simulink model "Tasks"  (R2024b)
settings: Solver=VariableStepAuto  StartTime=0.0  StopTime=3  RelTol=1e-3
model workspace (MATLAB code in the model file):
  | Ke = (2.53*10^(-3))*60/(2*pi); %V/(rad/s) Back EMF constant
  | Km = 24.2*10^(-3); %Nm/A    torque constant
  | L = 73*10^(-6); %H Terminal induction
  | R = 0.22; %ohm Terminal resictance
  | V = 24; %V Nominal supply voltage
  | J = 130*10^(-7);%kgm^2 %rotor inertia
  | frT = (7.72*10^(-7))*60/(2*pi); %Nm/(rad/s)  Friction torque dynamic
  | frTs=4.96e-3; %Nm Friction torque static
  | taum=4.9e-3; %Mechanical time constant
  | Mh=2635e-3; %Stall torqe Nm
  | I0=0.527; %no load current A
  | RADps_to_rpm=60/(2*pi);
  | RT=148e-3; %Rated torqe Nm
  | Rn=9650; %RPM rated speed
  | Rnnl=9700; %RPM rated speed no load
  | Mmaxout=55; %Max output torq
  | n=Mmaxout/Mh;
  | n1=n^0.5;
  | n2=n^0.5;
  | Jg1=6.5e-8;
  | Jg2=5.3e-8;
  | Jg=Jg1+(Jg2/(n1^2));
  | dj=1.5; %Nms/rad
  | 
  | dt=1.5; %Nms/rad
  | Kt=739; %Nm/rad
  | output_shaft_legth=(7.042+13.1+58)*(10^-3); %fyrkantstapp not included
  | avrage_diameter_output_shaft=(((24.5*10)+(19.6*11)+((58-19.6-24.5)*14)+(13.1*19.6)+(27.7*7.042))*(10^-6))/(output_shaft_legth); %fyrkantstapp not included.
  | input_shaft_solid_legth= (40.3-14)*10^-3;
  | avrage_diameter_input_solid_shaft= (((40.3-16.2)*5.9+(16.2-14)*11)*10^-6)/avrage_diameter_output_shaft;
  | input_shaft_hollow_legth=14e-3;
  | avrage_Odiameter_input_hollow_shaft=11e-3;
  | avrage_idiameter_input_hollow_shaft=8e-3;
  | Steel_density=7850; %kg/m^3
  | output_shaft_inertia=(Steel_density*output_shaft_legth*pi*((avrage_diameter_output_shaft/2)^4))/2;
  | input_shaft_solid_inertia=(Steel_density*input_shaft_solid_legth*pi*((avrage_diameter_input_solid_shaft/2)^4))/2;
  | input_shaft_hollow_inertia=(Steel_density*input_shaft_hollow_legth*pi*((avrage_Odiameter_input_hollow_shaft^2/4)-(avrage_idiameter_input_hollow_shaft^2/4)))*(((avrage_idiameter_input_hollow_shaft/2)^2)+((avrage_Odiameter_input_hollow_shaft/2)^2))/2;
  | input_shaft_inertia=input_shaft_hollow_inertia+input_shaft_solid_inertia;
  | Jin=input_shaft_inertia;
  | Jout=output_shaft_inertia;
  | J1=Jg+Jin+J;
  | J2=Jout;
  | A_Task6 =  [0, 0, 1, 0;
  |             0, 0, 0, 1;
  |             -Kt/(J1*n^2), Kt/(n*J1) , -(((dt/n^2)+(frT)+(Km*Ke/R))/J1),dt/(J1*n);
  |             Kt/(J2*n), -(Kt)/J2,dt/(n*J2), -(dj+dt)/J2];
  | B_Task6 = [0;
  |            0;
  |            Km/(R*J1);
  |            0];
  | C_Task6 = eye(4);
  | D_Task6 = [0;0;0;0];
  | 
  | 
  | 
  | Ks=4;%N/m
  | 
  | A_Task8 =  [0, 0, 1, 0;
  |             0, 0, 0, 1;
  |             -Kt/(J1*n^2), Kt/(n*J1) , -(((dt/n^2)+(frT)+(Km*Ke/R))/J1),dt/(J1*n);
  |             Kt/(J2*n), -(Kt+Ks)/J2,dt/(n*J2), -(dj+dt)/J2];
  | B_Task8 = [0;
  |            0;
  |            Km/(R*J1);
  |            0];
  | C_Task8 = eye(4);
  | D_Task8 = [0;0;0;0];
  | T=25;
  | Wtarget=3;
  | 
  | 
  | P=1.25e-3;%m
  | E=200e9; %Pa
  | Kj=Ks;
  | L0=100e-3; %m
  | sigmay=640e6; %Pa
  | %TargetT=(2*pi*L0*Kj*sigmay/(P*E));
  | r=4e-3; %m
  | Fy=pi*(r^2)*sigmay*10^6; %N
  | my=0.1;%-
  | Tmy=Fy*my*r; %Nm
  | thetay=(sigmay/((P/L0)*E))/(2*pi); %rad
  | Ftheta=(P/L0)*E*pi*(r^2)*2*pi*thetay*10^6; %F as a function of theta
  | Ty=Ks*thetay; %Nm
  | TargetT=Ty+Tmy; %Nm
  | 
  | 
  | Kpf=3/2.98;
undefined symbols (not defined in the file): sigbuilder_block
libraries: fl_lib x68, nesl_utility x18, slpidlib x5, sm_lib x4
(part 1 of 2)
settings Model: ParameterArgumentNames=A_Task6,A_Task8,B_Task6,B_Task8,C_Task6,C_Task8,D_Task6,D_Task8,I0,J,J1,J2,Jg,Jg1,Jg2,Jin,Jout,Ke,Km,Ks,Kt,L,Mh,Mmaxout,R,RADps_to_rpm,RT,Rn,Rnnl,Steel_density,T,V,Wtarget,avrage_Odiameter_input_hollow_shaft,avrage_diameter_input_solid_shaft,avrage_diameter_output_shaft,avrage_idiameter_input_hollow_shaft,dj,dt,frT,frTs,input_shaft_hollow_inertia,input_shaft_hollow_legth,input_shaft_inertia,input_shaft_solid_inertia,input_shaft_solid_legth,n,n1,n2,output_shaft_inertia,output_shaft_legth,taum  Creator=Johki  LastModifiedBy=chienh1

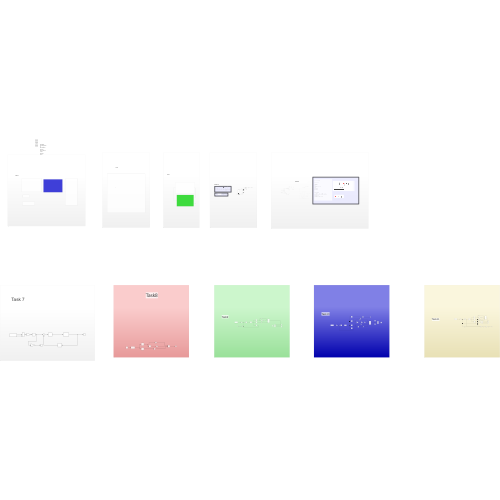
[thumbnail: Simulink's stored preview of the top-level diagram]
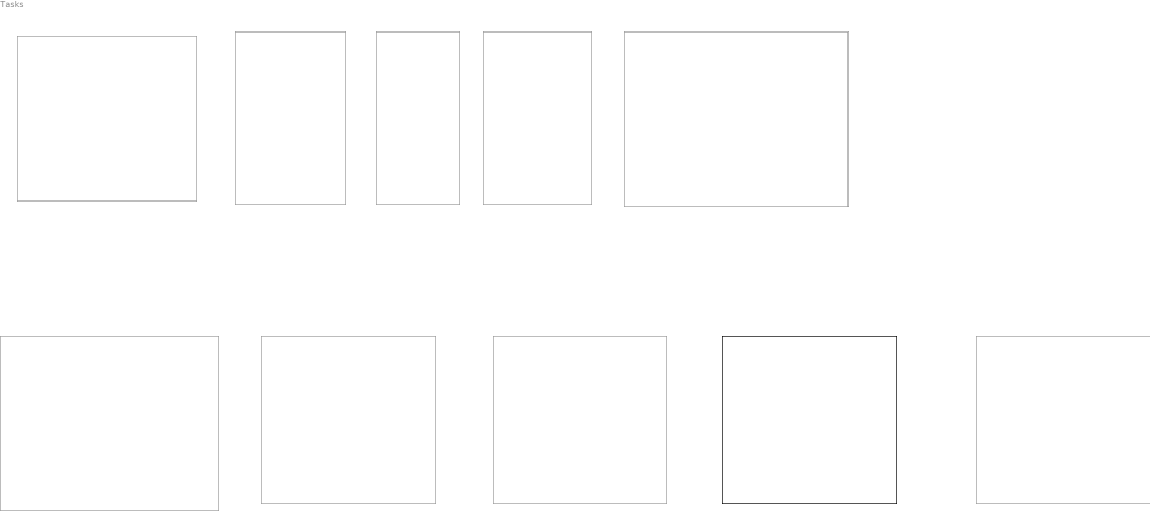
== system Tasks ==
  note: 2024-09-24:
      | Done: Repport so far
      | Start: Task9-11
      |
      | 2024-10-1
      | Done: Task9-11
      | Finnish
      |
      | 2024-10-7
      | "Done"
  note: 1: 8 points,
      | 2: 4 points,
      | 3: 4 points,
      | 4: 6 points,
      | 5: 2 points,
      | 6: 16 points,
      | 7: 6 points,
      | 8: 6 points,
      | 9: 8 points,
      | 10: 6 points,
      | 11: 4 points .
  Subsystem : Subsystem  Commented=on
  Subsystem1 : Subsystem  Commented=on
  Subsystem2 : Subsystem  Commented=on
  Subsystem3 : Subsystem  Commented=on
  Subsystem4 : Subsystem  Commented=on
  Subsystem5 : Subsystem  Commented=on
  Subsystem6 : Subsystem  Commented=on
  Subsystem7 : Subsystem
  Subsystem8 : Subsystem  Commented=on
  "Task6 " : Subsystem  Commented=on

== system Tasks/Subsystem ==
  note: Task 3
  Block diagram : Subsystem
  PI controller : Subsystem
  Terminator : Terminator
  wires:
  Block diagram/1(W) -> PI controller/1(ang velocity)
  PI controller/1(V) -> Block diagram/1(V)
  Block diagram/2(rpm) -> Terminator/1  "RPM_Block_dig"

== system Tasks/Subsystem1 ==
  note: Task 1
  Block diagram1 : Subsystem  Commented=on
  "SD " : Subsystem  Commented=on
  "Simscape " : Subsystem  Commented=on
  Simulink Model via State-Space Representation : Subsystem  Commented=on
  "Simulink Model via Transfer Function " : Subsystem  Commented=on

== system Tasks/Subsystem2 ==
  note: Task 2
  Subsystem5 : Subsystem
  Terminator3 : Terminator

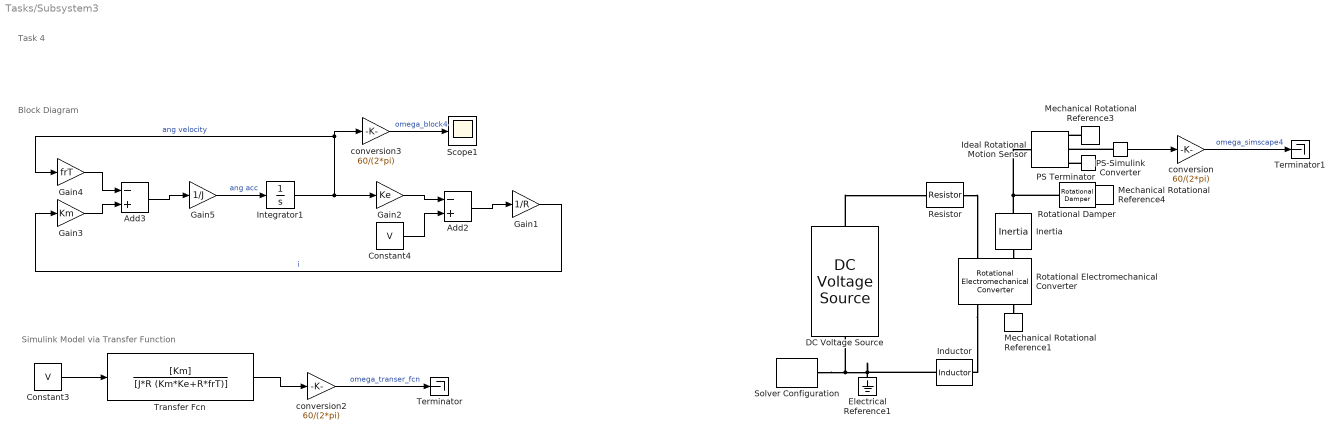
== system Tasks/Subsystem3 ==
  note: Block Diagram
  note: Simulink Model via Transfer Function
  note: Task 4
  Add2 : Sum  Inputs=-+
  Add3 : Sum  Inputs=-+
  Constant3 : Constant  Value=V
  Constant4 : Constant  Value=V
  DC Voltage Source : fl_lib/Electrical/Electrical Sources/DC Voltage Source  v0=V V
  Electrical Reference1 : fl_lib/Electrical/Electrical Elements/Electrical Reference
  Gain1 : Gain  Gain=1/R
  Gain2 : Gain  Gain=Ke
  Gain3 : Gain  Gain=Km
  Gain4 : Gain  Gain=frT
  Gain5 : Gain  Gain=1/J
  Ideal Rotational Motion Sensor : fl_lib/Mechanical/Mechanical Sensors/Ideal Rotational Motion Sensor  reference=foundation.enum.MeasurementReference.difference  acceleration_port=false  velocity_port=true  position_port=true  wrap_angle=simscape.enum.onoff.off  offset=0 rad
  Inductor : fl_lib/Electrical/Electrical Elements/Inductor  l=L H  r=0 Ohm  g=0 1/Ohm  i_specify=off  i_priority=None  i=0 A  i_nominal_specify=off  i_nominal_value=1  i_nominal_unit=A  v_specify=off  v_priority=None  v=0 V  v_nominal_specify=off  v_nominal_value=1  v_nominal_unit=V  i_L_specify=off  i_L_priority=High  i_L=0 A  i_L_nominal_specify=off  i_L_nominal_value=1  i_L_nominal_unit=A
  Inertia : fl_lib/Mechanical/Rotational Elements/Inertia  inertia=J kg*m^2  num_ports=foundation.enum.numPorts2.two  w_specify=off  w_priority=High  w=0 rad/s  w_nominal_specify=off  w_nominal_value=1  w_nominal_unit=rad/s  t_specify=off  t_priority=None  t=0 N*m  t_nominal_specify=off  t_nominal_value=1  t_nominal_unit=N*m
      settings: InternalSimscapePortConfiguration="{\"Bottom\":[],\"Left\":[{\"id\":\"I\",\"label\":\"\",\"type\":\"foundation.mechanical.rotational.rotational\"}],\"Right\":[{\"id\":\"J\",\"label\":\"\",\"type\":\"foundation.mechanical.rotational.rotational\"}],\"Top\":[]}"
  Integrator1 : Integrator
  Mechanical Rotational Reference1 : fl_lib/Mechanical/Rotational Elements/Mechanical Rotational Reference
  Mechanical Rotational Reference3 : fl_lib/Mechanical/Rotational Elements/Mechanical Rotational Reference
  Mechanical Rotational Reference4 : fl_lib/Mechanical/Rotational Elements/Mechanical Rotational Reference
  PS Terminator : fl_lib/Physical Signals/Sinks/PS Terminator
  PS-Simulink Converter : nesl_utility/PS-Simulink Converter  PhysicalDomain=network_engine_domain  SubClassName=ps_output  LeftPortType=input  RightPortType=output  PseudoPeriodic=off  Frequencies=[]  VectorFormat=inherit  Unit=inherit  AffineConversion=off
  Resistor : fl_lib/Electrical/Electrical Elements/Resistor  R=R Ohm  i_specify=off  i_priority=None  i=0 A  i_nominal_specify=off  i_nominal_value=1  i_nominal_unit=A  v_specify=off  v_priority=None  v=0 V  v_nominal_specify=off  v_nominal_value=1  v_nominal_unit=V
  Rotational Electromechanical Converter : fl_lib/Electrical/Electrical Elements/Rotational Electromechanical Converter  K=Ke V*s/rad  i_specify=off  i_priority=None  i=0 A  i_nominal_specify=off  i_nominal_value=1  i_nominal_unit=A  v_specify=off  v_priority=None  v=0 V  v_nominal_specify=off  v_nominal_value=1  v_nominal_unit=V  t_specify=off  t_priority=None  t=0 N*m  t_nominal_specify=off  t_nominal_value=1  t_nominal_unit=N*m  w_specify=on  w_priority=None  w=0 rad/s  w_nominal_specify=off  w_nominal_value=1  w_nominal_unit=rad/s
  Rotational Damper : fl_lib/Mechanical/Rotational Elements/Rotational Damper  D=frT N*m*s/rad  w_specify=off  w_priority=None  w=0 rad/s  w_nominal_specify=off  w_nominal_value=1  w_nominal_unit=rad/s  t_specify=off  t_priority=None  t=0 N*m  t_nominal_specify=off  t_nominal_value=1  t_nominal_unit=N*m
  Scope1 : Scope
  Solver Configuration : nesl_utility/Solver Configuration  PhysicalDomain=network_engine_domain  SubClassName=solver  LeftPortType=input  RightPortType=generic  Tones=[]  Harmonics=[]  SimulateNoise=off  Profile=off  UseLocalSampling=off  EnableSwitchedLinearOptims=on  FrequencyDomain=off  UseCCode=off  RelTol=0.001  AbsTol=0.001  MinStep=1e-09  ToWorkspace=off  RevertToSquareIcSolve=off  NumHomotopyIterations=100  PhasorMode=off  PhasorModeNumHarmonics=1  ConsistencySolver=NEWTON_FTOL  IndexReductionMethod=DerivativeReplacement  DoDC=off  ResidualTolerance=1e-09  ConsistencyTolSource=GLOBAL  ConsistencyAbsTol=0.001  ConsistencyRelTol=0.001  ConsistencyTolFactor=0.001  UseLocalSolver=off  LocalSolverChoice=NE_BACKWARD_EULER_ADVANCER  ResolveIndetEquations=on  FunctionEvalNumThread=1  LocalSolverSampleTime=0.001  DoFixedCost=off  MaxNonlinIter=3  MaxModeIter=2  ComputeImpulses=off  ImpulseIterations=2  LinearAlgebra=auto  LinearAlgebraNumThread=0  EquationFormulation=NE_TIME_EF  DelaysMemoryBudget=1024  AutomaticFiltering=on  FilteringTimeConstant=0.001  PartitionStorageMethod=AS_NEEDED  PartitionMemoryBudget=1024  PartitionMethod=ROBUST  MultibodyUseLocalSolver=off  MultibodyLocalSolverChoice=ODE1  MultibodyLocalSolverSampleTime=0.001
  Terminator : Terminator
  Terminator1 : Terminator
  Transfer Fcn : TransferFcn  Numerator=[Km]  Denominator=[J*R (Km*Ke+R*frT)]
  conversion : Gain  Gain=60/(2*pi)
  conversion2 : Gain  Gain=60/(2*pi)
  conversion3 : Gain  Gain=60/(2*pi)
  wires:
  Constant3/1 -> Transfer Fcn/1
  Transfer Fcn/1 -> conversion2/1
  conversion2/1 -> Terminator/1  "omega_transer_fcn"
  Gain2/1 -> Add2/1
  Add2/1 -> Gain1/1
  Gain1/1 -> Gain3/1  "i"
  Gain4/1 -> Add3/1
  Integrator1/1 -> conversion3/1, Gain4/1, Gain2/1  "ang velocity"
  Add3/1 -> Gain5/1
  Gain5/1 -> Integrator1/1  "ang acc"
  Constant4/1 -> Add2/2
  conversion3/1 -> Scope1/1  "omega_block4"
  Gain3/1 -> Add3/2
  conversion/1 -> Terminator1/1  "omega_simscape4"
  PS-Simulink Converter/1 -> conversion/1
  connections:
  DC Voltage Source/RConn1 -- Solver Configuration/RConn1 -- Inductor/RConn1 -- Electrical Reference1/LConn1
  Inertia/LConn1 -- Rotational Damper/LConn1 -- Ideal Rotational Motion Sensor/LConn1
  DC Voltage Source/LConn1 -- Resistor/LConn1
  PS-Simulink Converter/LConn1 -- Ideal Rotational Motion Sensor/RConn2
  Inertia/RConn1 -- Rotational Electromechanical Converter/LConn2
  Rotational Electromechanical Converter/RConn1 -- Inductor/LConn1
  Mechanical Rotational Reference4/LConn1 -- Rotational Damper/RConn1
  Rotational Electromechanical Converter/RConn2 -- Mechanical Rotational Reference1/LConn1
  Mechanical Rotational Reference3/LConn1 -- Ideal Rotational Motion Sensor/RConn1
  PS Terminator/LConn1 -- Ideal Rotational Motion Sensor/RConn3
  Resistor/RConn1 -- Rotational Electromechanical Converter/LConn1

== system Tasks/Subsystem4 ==
  note: Task 7
  Acceleration ref. : Subsystem  Tag=STV Subsys  LoadFcn=sigbuilder_block('load');  StartFcn=sigbuilder_block('start');  StopFcn=sigbuilder_block('stop');  ClipboardFcn=sigbuilder_block('clipboard');  mask(Sigbuilder block){tuvar=[0:10]}
      mask help: Sigbuilder GUI
      mask init:
      | if ~strcmp(get_param(bdroot(gcbh),'SimulationStatus'),'stopped') tuvar = sigbuilder_block('maskInit'); end
      settings: CopyFcn=sigbuilder_block('copy');  DeleteFcn=sigbuilder_block('delete');  ModelCloseFcn=sigbuilder_block('modelClose');  PreSaveFcn=sigbuilder_block('preSave');  PauseFcn=sigbuilder_block('pause')  ContinueFcn=sigbuilder_block('continue')  NameChangeFcn=sigbuilder_block('namechange');  OpenFcn=sigbuilder_block('open',[214.5 118 550.5 362 ]);  CloseFcn=sigbuilder_block('close');
      mask Display: plot(0, 0, 100, 100,[2, 2, 32, 32, 2], [68, 8, 8, 68, 68],[32, 2], [38, 38], [32, 19, 2],[53, 60, 44], [32, 17, 17, 2],[16, 16, 31, 31]);txt = getActiveGroup(gcbh);text(2, 100, txt,'verticalAlignment', 'top');
  PID Controller : slpidlib/PID Controller  Controller=PI  Form=Parallel  TimeDomain=Continuous-time  UseExternalTs=off  SampleTime=-1  IntegratorMethod=Forward Euler  FilterMethod=Forward Euler  ControllerParametersSource=internal  P=1.2  I=51  UseKiTs=off  D=0  UseExternalDerivativeSource=off  N=100  UseFilter=on  TunerSelectOption=Transfer Function Based (PID Tuner App)  InitialConditionSource=internal  InitialConditionForIntegrator=0  InitialConditionForFilter=0  DifferentiatorICPrevScaledInput=0  ExternalReset=none  TrackingMode=off  Kt=1  LimitOutput=off  SatLimitsSource=internal  UpperSaturationLimit=24  LowerSaturationLimit=0  LinearizeAsGain=on  AntiWindupMode=none  Kb=1  LimitIntegrator=off  UpperIntegratorSaturationLimit=inf  LowerIntegratorSaturationLimit=-inf  POutMin=[]  POutMax=[]  IOutMin=[]  IOutMax=[]  DOutMin=[]  DOutMax=[]  NOutMin=[]  NOutMax=[]  SumOutMin=[]  SumOutMax=[]  SaturationOutMin=[]  SaturationOutMax=[]  PParamMin=[]  PParamMax=[]  IParamMin=[]  IParamMax=[]  DParamMin=[]  DParamMax=[]  NParamMin=[]  NParamMax=[]  KbParamMin=[]  KbParamMax=[]  KtParamMin=[]  KtParamMax=[]  KbOutMin=[]  KbOutMax=[]  KtOutMin=[]  KtOutMax=[]  IntegratorOutMin=[]  IntegratorOutMax=[]  FilterOutMin=[]  FilterOutMax=[]  SumI1OutMin=[]  SumI1OutMax=[]  SumI2OutMin=[]  SumI2OutMax=[]  SumI3OutMin=[]  SumI3OutMax=[]  SumI4OutMin=[]  SumI4OutMax=[]  SumDOutMin=[]  SumDOutMax=[]  DifferentiatorOutMin=[]  DifferentiatorOutMax=[]  FilterDiffOutCoefMin=[]  FilterDiffOutCoefMax=[]  ReciprocalOutMin=[]  ReciprocalOutMax=[]  SumDenOutMin=[]  SumDenOutMax=[]  SumNumOutMin=[]  SumNumOutMax=[]  DivideOutMin=[]  DivideOutMax=[]  UdiffTsProdOutMin=[]  UdiffTsProdOutMax=[]  NTsProdOutMin=[]  NTsProdOutMax=[]  UintegralTsProdOutMin=[]  UintegralTsProdOutMax=[]  UngainTsProdOutMin=[]  UngainTsProdOutMax=[]  ClampingZeroOutDataTypeStr=Inherit: Inherit via back propagation  ClampingZeroOutMin=[]  ClampingZeroOutMax=[]  FilterDenConstantOutDataTypeStr=Inherit: Inherit via back propagation  FilterDenConstantOutMin=[]  FilterDenConstantOutMax=[]  PCopyOutDataTypeStr=Inherit: Inherit via back propagation  PCopyOutMin=[]  PCopyOutMax=[]  NCopyOutDataTypeStr=Inherit: Inherit via back propagation  NCopyOutMin=[]  NCopyOutMax=[]  IntegratorContinuousStateAttributes=''  IntegratorStateMustResolveToSignalObject=off  IntegratorRTWStateStorageClass=Auto  FilterContinuousStateAttributes=''  FilterStateMustResolveToSignalObject=off  FilterRTWStateStorageClass=Auto  ParallelPVariant=InternalParameters  IdealPVariant=Disabled  IVariant=InternalParameters  DVariant=Disabled  IntegratorVariant=Continuous  SatVariant=Disabled  AWVariant=Passthrough  PCopyVariant=Disabled  TRVariant=Disabled  FdbkBlocksVariant=Forward  IdealPFdbkVariant=Disabled  SatFdbkVariant=Disabled  DerivativeFilterVariant=Disabled  NVariant=Disabled  NCopyVariant=Disabled_SignalSpec  FilterICVariant=Disabled  IntegratorICVariant=InternalICs  ExternalResetVariant=Disabled  TRSumVariant=Passthrough  SumFdbkVariant=Disabled  SumVariant=Sum_PI  TsampFilterVariant=InternalTs  TsampNgainVariant=Passthrough  TsampIntegralVariant=Disabled_SignalSpec  ExternalSaturationOutDataTypeStr=Inherit: Same as second input  DerivativeSourceVariant=Disabled  PreIntVariant=InternalPreInt
  Scaling factor : Gain  Gain=15*n
  Scaling factor2 : Gain  Gain=1/n
  Selector : Selector  IndexMode=Zero-based  InputPortWidth=4  IndexOptions=Index vector (dialog)  Indices=2  OutputSizes=1
  State-Space : StateSpace  A=A_Task6  B=B_Task6  C=C_Task6  D=D_Task6  InitialCondition=0
  Sum : Sum  Inputs=|+-
  Sum2 : Sum  Inputs=|++
  Terminator : Terminator
  Vellocity ref : Integrator
  Y : Terminator
  wires:
  Sum2/1 -> Scaling factor/1
  Scaling factor/1 -> Vellocity ref/1
  Acceleration ref./1(Signal 1) -> Sum2/1
  Acceleration ref./2(Signal 2) -> Sum2/2
  State-Space/1 -> Y/1, Selector/1  "Y Task7"
  Sum/1 -> PID Controller/1
  Vellocity ref/1 -> Scaling factor2/1, Sum/1
  Selector/1 -> Sum/2  "phi1_dot_task7"
  PID Controller/1 -> State-Space/1  "V_Task7"
  Scaling factor2/1 -> Terminator/1  "Ref nut speed"

== system Tasks/Subsystem5 ==
  note: Task8
  24 V : Constant  Value=V
  Add : Sum  Inputs=+++
  Derivative : Derivative
  Gain : Gain  Gain=Ks
  Gain1 : Gain  Gain=dj
  Gain2 : Gain  Gain=J2
  Selector : Selector  InputPortWidth=4  IndexOptions=Index vector (dialog)  Indices=2  OutputSizes=1
  Selector1 : Selector  InputPortWidth=4  IndexOptions=Index vector (dialog)  Indices=4  OutputSizes=1
  State-Space : StateSpace  A=A_Task8  B=B_Task8  C=C_Task8  D=D_Task8  InitialCondition=0
  Terminator : Terminator
  wires:
  24 V/1 -> State-Space/1
  State-Space/1 -> Selector1/1, Selector/1  "States Task8"
  Selector/1 -> Gain/1  "phi 2"
  Selector1/1 -> Gain1/1, Derivative/1  "phi2 dot"
  Derivative/1 -> Gain2/1  "phi2 dotdot"
  Gain2/1 -> Add/2  "torsional inertia"
  Gain1/1 -> Add/1  "damping torque"
  Gain/1 -> Add/3  "torsional spring torque"
  Add/1 -> Terminator/1  "Total torque"

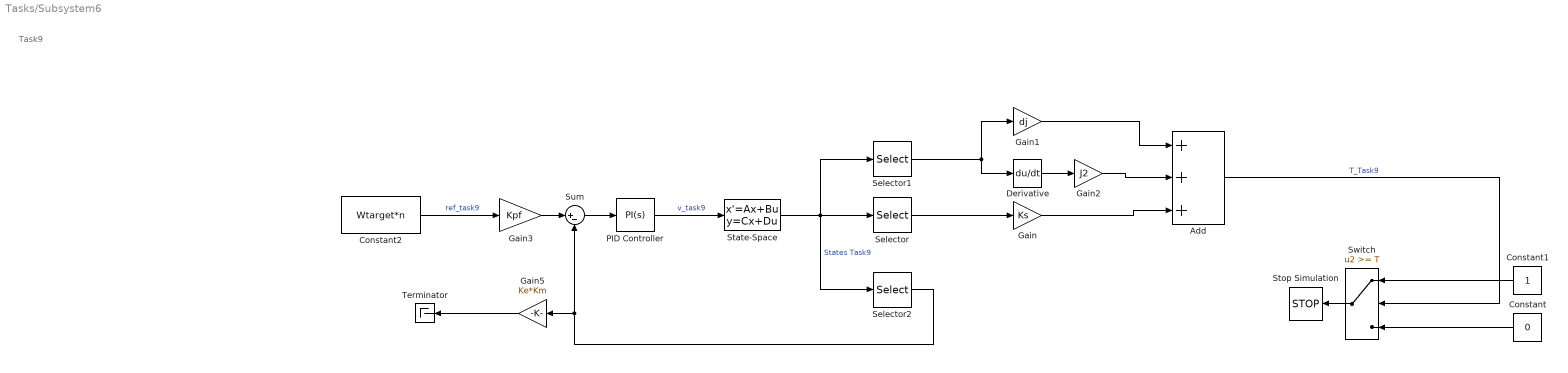
== system Tasks/Subsystem6 ==
  note: Task9
  Add : Sum  Inputs=+++
  Constant : Constant  Value=0
  Constant1 : Constant
  Constant2 : Constant  Value=Wtarget*n  VectorParams1D=off
  Derivative : Derivative
  Gain : Gain  Gain=Ks
  Gain1 : Gain  Gain=dj
  Gain2 : Gain  Gain=J2
  Gain3 : Gain  Gain=Kpf
  Gain5 : Gain  Gain=Ke*Km
  PID Controller : slpidlib/PID Controller  Controller=PI  Form=Parallel  TimeDomain=Continuous-time  UseExternalTs=off  SampleTime=-1  IntegratorMethod=Forward Euler  FilterMethod=Forward Euler  ControllerParametersSource=internal  P=24/(Wtarget*n*(Kpf))  I=1200  UseKiTs=off  D=0  UseExternalDerivativeSource=off  N=100  UseFilter=on  TunerSelectOption=Transfer Function Based (PID Tuner App)  InitialConditionSource=internal  InitialConditionForIntegrator=0  InitialConditionForFilter=0  DifferentiatorICPrevScaledInput=0  ExternalReset=none  TrackingMode=off  Kt=1  LimitOutput=off  SatLimitsSource=internal  UpperSaturationLimit=24  LowerSaturationLimit=0  LinearizeAsGain=on  AntiWindupMode=none  Kb=1  LimitIntegrator=off  UpperIntegratorSaturationLimit=inf  LowerIntegratorSaturationLimit=-inf  POutMin=[]  POutMax=[]  IOutMin=[]  IOutMax=[]  DOutMin=[]  DOutMax=[]  NOutMin=[]  NOutMax=[]  SumOutMin=[]  SumOutMax=[]  SaturationOutMin=[]  SaturationOutMax=[]  PParamMin=[]  PParamMax=[]  IParamMin=[]  IParamMax=[]  DParamMin=[]  DParamMax=[]  NParamMin=[]  NParamMax=[]  KbParamMin=[]  KbParamMax=[]  KtParamMin=[]  KtParamMax=[]  KbOutMin=[]  KbOutMax=[]  KtOutMin=[]  KtOutMax=[]  IntegratorOutMin=[]  IntegratorOutMax=[]  FilterOutMin=[]  FilterOutMax=[]  SumI1OutMin=[]  SumI1OutMax=[]  SumI2OutMin=[]  SumI2OutMax=[]  SumI3OutMin=[]  SumI3OutMax=[]  SumI4OutMin=[]  SumI4OutMax=[]  SumDOutMin=[]  SumDOutMax=[]  DifferentiatorOutMin=[]  DifferentiatorOutMax=[]  FilterDiffOutCoefMin=[]  FilterDiffOutCoefMax=[]  ReciprocalOutMin=[]  ReciprocalOutMax=[]  SumDenOutMin=[]  SumDenOutMax=[]  SumNumOutMin=[]  SumNumOutMax=[]  DivideOutMin=[]  DivideOutMax=[]  UdiffTsProdOutMin=[]  UdiffTsProdOutMax=[]  NTsProdOutMin=[]  NTsProdOutMax=[]  UintegralTsProdOutMin=[]  UintegralTsProdOutMax=[]  UngainTsProdOutMin=[]  UngainTsProdOutMax=[]  ClampingZeroOutDataTypeStr=Inherit: Inherit via back propagation  ClampingZeroOutMin=[]  ClampingZeroOutMax=[]  FilterDenConstantOutDataTypeStr=Inherit: Inherit via back propagation  FilterDenConstantOutMin=[]  FilterDenConstantOutMax=[]  PCopyOutDataTypeStr=Inherit: Inherit via back propagation  PCopyOutMin=[]  PCopyOutMax=[]  NCopyOutDataTypeStr=Inherit: Inherit via back propagation  NCopyOutMin=[]  NCopyOutMax=[]  IntegratorContinuousStateAttributes=''  IntegratorStateMustResolveToSignalObject=off  IntegratorRTWStateStorageClass=Auto  FilterContinuousStateAttributes=''  FilterStateMustResolveToSignalObject=off  FilterRTWStateStorageClass=Auto  ParallelPVariant=InternalParameters  IdealPVariant=Disabled  IVariant=InternalParameters  DVariant=Disabled  IntegratorVariant=Continuous  SatVariant=Disabled  AWVariant=Passthrough  PCopyVariant=Disabled  TRVariant=Disabled  FdbkBlocksVariant=Forward  IdealPFdbkVariant=Disabled  SatFdbkVariant=Disabled  DerivativeFilterVariant=Disabled  NVariant=Disabled  NCopyVariant=Disabled_SignalSpec  FilterICVariant=Disabled  IntegratorICVariant=InternalICs  ExternalResetVariant=Disabled  TRSumVariant=Passthrough  SumFdbkVariant=Disabled  SumVariant=Sum_PI  TsampFilterVariant=InternalTs  TsampNgainVariant=Passthrough  TsampIntegralVariant=Disabled_SignalSpec  ExternalSaturationOutDataTypeStr=Inherit: Same as second input  DerivativeSourceVariant=Disabled  PreIntVariant=InternalPreInt
  Selector : Selector  InputPortWidth=4  IndexOptions=Index vector (dialog)  Indices=2  OutputSizes=1
  Selector1 : Selector  InputPortWidth=4  IndexOptions=Index vector (dialog)  Indices=4  OutputSizes=1
  Selector2 : Selector  InputPortWidth=4  IndexOptions=Index vector (dialog)  Indices=3  OutputSizes=1
  State-Space : StateSpace  A=A_Task8  B=B_Task8  C=C_Task8  D=D_Task8  InitialCondition=0
  Stop Simulation : Stop
  Sum : Sum  Inputs=|+-
  Switch : Switch  Threshold=T  SaturateOnIntegerOverflow=off  InputSameDT=off
  Terminator : Terminator
  wires:
  Switch/1 -> Stop Simulation/1
  Constant/1 -> Switch/3
  Constant1/1 -> Switch/1
  Selector1/1 -> Derivative/1, Gain1/1
  Selector/1 -> Gain/1
  State-Space/1 -> Selector2/1, Selector/1, Selector1/1  "States Task9"
  Derivative/1 -> Gain2/1
  Add/1 -> Switch/2  "T_Task9"
  Gain/1 -> Add/3
  PID Controller/1 -> State-Space/1  "v_task9"
  Sum/1 -> PID Controller/1
  Selector2/1 -> Gain5/1, Sum/2
  Constant2/1 -> Gain3/1  "ref_task9"
  Gain3/1 -> Sum/1
  Gain2/1 -> Add/2
  Gain1/1 -> Add/1
  Gain5/1 -> Terminator/1

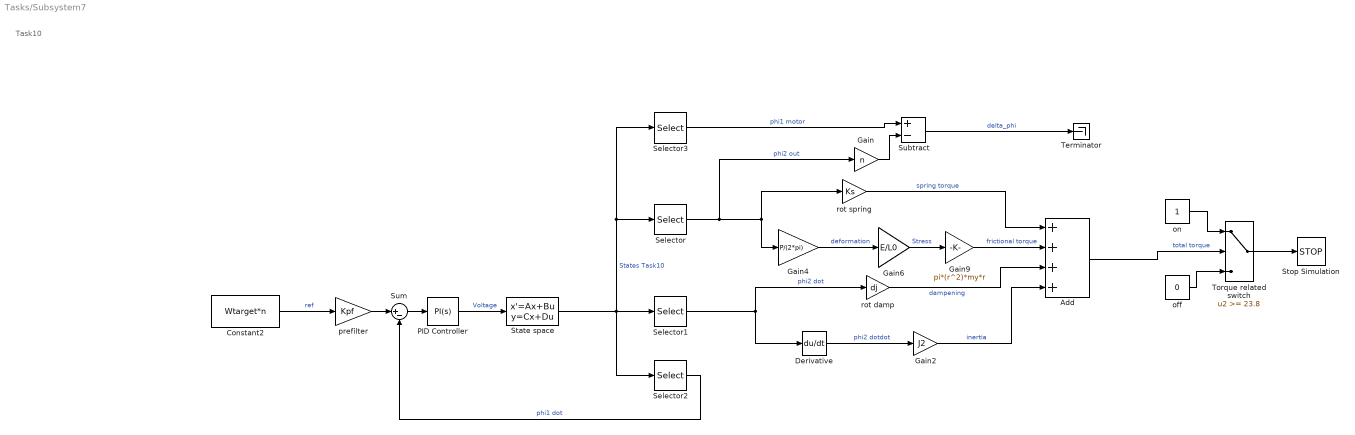
== system Tasks/Subsystem7 ==
  note: Task10
  Add : Sum  Inputs=++++
  Constant2 : Constant  Value=Wtarget*n  VectorParams1D=off
  Derivative : Derivative
  Gain : Gain  Gain=n
  Gain2 : Gain  Gain=J2
  Gain4 : Gain  Gain=P/(2*pi)
  Gain6 : Gain  Gain=E/L0
  Gain9 : Gain  Gain=pi*(r^2)*my*r
  PID Controller : slpidlib/PID Controller  Controller=PI  Form=Parallel  TimeDomain=Continuous-time  UseExternalTs=off  SampleTime=-1  IntegratorMethod=Forward Euler  FilterMethod=Forward Euler  ControllerParametersSource=internal  P=24/(Wtarget*n*Kpf)  I=1200  UseKiTs=off  D=0  UseExternalDerivativeSource=off  N=100  UseFilter=on  TunerSelectOption=Transfer Function Based (PID Tuner App)  InitialConditionSource=internal  InitialConditionForIntegrator=0  InitialConditionForFilter=0  DifferentiatorICPrevScaledInput=0  ExternalReset=none  TrackingMode=off  Kt=1  LimitOutput=off  SatLimitsSource=internal  UpperSaturationLimit=24  LowerSaturationLimit=0  LinearizeAsGain=on  AntiWindupMode=none  Kb=1  LimitIntegrator=off  UpperIntegratorSaturationLimit=inf  LowerIntegratorSaturationLimit=-inf  POutMin=[]  POutMax=[]  IOutMin=[]  IOutMax=[]  DOutMin=[]  DOutMax=[]  NOutMin=[]  NOutMax=[]  SumOutMin=[]  SumOutMax=[]  SaturationOutMin=[]  SaturationOutMax=[]  PParamMin=[]  PParamMax=[]  IParamMin=[]  IParamMax=[]  DParamMin=[]  DParamMax=[]  NParamMin=[]  NParamMax=[]  KbParamMin=[]  KbParamMax=[]  KtParamMin=[]  KtParamMax=[]  KbOutMin=[]  KbOutMax=[]  KtOutMin=[]  KtOutMax=[]  IntegratorOutMin=[]  IntegratorOutMax=[]  FilterOutMin=[]  FilterOutMax=[]  SumI1OutMin=[]  SumI1OutMax=[]  SumI2OutMin=[]  SumI2OutMax=[]  SumI3OutMin=[]  SumI3OutMax=[]  SumI4OutMin=[]  SumI4OutMax=[]  SumDOutMin=[]  SumDOutMax=[]  DifferentiatorOutMin=[]  DifferentiatorOutMax=[]  FilterDiffOutCoefMin=[]  FilterDiffOutCoefMax=[]  ReciprocalOutMin=[]  ReciprocalOutMax=[]  SumDenOutMin=[]  SumDenOutMax=[]  SumNumOutMin=[]  SumNumOutMax=[]  DivideOutMin=[]  DivideOutMax=[]  UdiffTsProdOutMin=[]  UdiffTsProdOutMax=[]  NTsProdOutMin=[]  NTsProdOutMax=[]  UintegralTsProdOutMin=[]  UintegralTsProdOutMax=[]  UngainTsProdOutMin=[]  UngainTsProdOutMax=[]  ClampingZeroOutDataTypeStr=Inherit: Inherit via back propagation  ClampingZeroOutMin=[]  ClampingZeroOutMax=[]  FilterDenConstantOutDataTypeStr=Inherit: Inherit via back propagation  FilterDenConstantOutMin=[]  FilterDenConstantOutMax=[]  PCopyOutDataTypeStr=Inherit: Inherit via back propagation  PCopyOutMin=[]  PCopyOutMax=[]  NCopyOutDataTypeStr=Inherit: Inherit via back propagation  NCopyOutMin=[]  NCopyOutMax=[]  IntegratorContinuousStateAttributes=''  IntegratorStateMustResolveToSignalObject=off  IntegratorRTWStateStorageClass=Auto  FilterContinuousStateAttributes=''  FilterStateMustResolveToSignalObject=off  FilterRTWStateStorageClass=Auto  ParallelPVariant=InternalParameters  IdealPVariant=Disabled  IVariant=InternalParameters  DVariant=Disabled  IntegratorVariant=Continuous  SatVariant=Disabled  AWVariant=Passthrough  PCopyVariant=Disabled  TRVariant=Disabled  FdbkBlocksVariant=Forward  IdealPFdbkVariant=Disabled  SatFdbkVariant=Disabled  DerivativeFilterVariant=Disabled  NVariant=Disabled  NCopyVariant=Disabled_SignalSpec  FilterICVariant=Disabled  IntegratorICVariant=InternalICs  ExternalResetVariant=Disabled  TRSumVariant=Passthrough  SumFdbkVariant=Disabled  SumVariant=Sum_PI  TsampFilterVariant=InternalTs  TsampNgainVariant=Passthrough  TsampIntegralVariant=Disabled_SignalSpec  ExternalSaturationOutDataTypeStr=Inherit: Same as second input  DerivativeSourceVariant=Disabled  PreIntVariant=InternalPreInt
  Selector : Selector  InputPortWidth=4  IndexOptions=Index vector (dialog)  Indices=2  OutputSizes=1
  Selector1 : Selector  InputPortWidth=4  IndexOptions=Index vector (dialog)  Indices=4  OutputSizes=1
  Selector2 : Selector  InputPortWidth=4  IndexOptions=Index vector (dialog)  Indices=3  OutputSizes=1
  Selector3 : Selector  InputPortWidth=4  IndexOptions=Index vector (dialog)  Indices=1  OutputSizes=1
  State space : StateSpace  A=A_Task8  B=B_Task8  C=C_Task8  D=D_Task8  InitialCondition=0
  Stop Simulation : Stop
  Subtract : Sum  Inputs=+-
  Sum : Sum  Inputs=|+-
  Terminator : Terminator
  Torque related switch : Switch  Threshold=23.8  SaturateOnIntegerOverflow=off  InputSameDT=off
  off : Constant  Value=0
  on : Constant
  prefilter : Gain  Gain=Kpf
  rot damp : Gain  Gain=dj
  rot spring : Gain  Gain=Ks
  wires:
  Selector2/1 -> Sum/2  "phi1 dot"
  prefilter/1 -> Sum/1
  Constant2/1 -> prefilter/1  "ref"
  Gain2/1 -> Add/4  "inertia"
  Torque related switch/1 -> Stop Simulation/1
  rot spring/1 -> Add/1  "spring torque"
  PID Controller/1 -> State space/1  "Voltage"
  Sum/1 -> PID Controller/1
  Add/1 -> Torque related switch/2  "total torque"
  State space/1 -> Selector3/1, Selector/1, Selector1/1, Selector2/1  "States Task10"
  Derivative/1 -> Gain2/1  "phi2 dotdot"
  off/1 -> Torque related switch/3
  on/1 -> Torque related switch/1
  rot damp/1 -> Add/3  "dampening"
  Selector1/1 -> rot damp/1, Derivative/1  "phi2 dot"
  Gain4/1 -> Gain6/1  "deformation"
  Gain6/1 -> Gain9/1  "Stress"
  Selector/1 -> Gain4/1, rot spring/1, Gain/1  "phi2 out"
  Gain9/1 -> Add/2  "frictional torque"
  Subtract/1 -> Terminator/1  "delta_phi"
  Selector3/1 -> Subtract/1  "phi1 motor"
  Gain/1 -> Subtract/2

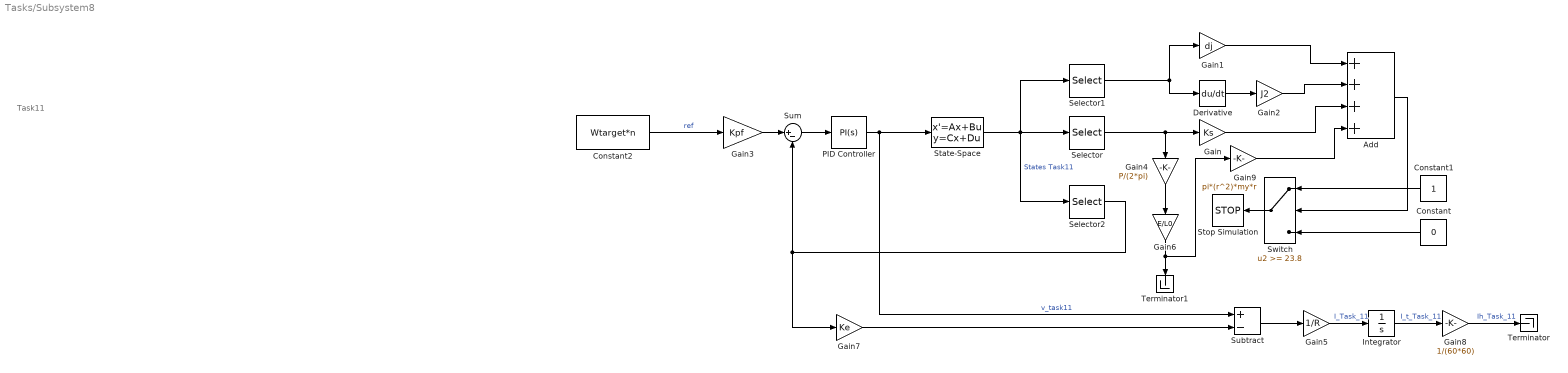
== system Tasks/Subsystem8 ==
  note: Task11
  Add : Sum  Inputs=++++
  Constant : Constant  Value=0
  Constant1 : Constant
  Constant2 : Constant  Value=Wtarget*n  VectorParams1D=off
  Derivative : Derivative
  Gain : Gain  Gain=Ks
  Gain1 : Gain  Gain=dj
  Gain2 : Gain  Gain=J2
  Gain3 : Gain  Gain=Kpf
  Gain4 : Gain  Gain=P/(2*pi)
  Gain5 : Gain  Gain=1/R
  Gain6 : Gain  Gain=E/L0
  Gain7 : Gain  Gain=Ke
  Gain8 : Gain  Gain=1/(60*60)
  Gain9 : Gain  Gain=pi*(r^2)*my*r
  Integrator : Integrator
  PID Controller : slpidlib/PID Controller  Controller=PI  Form=Parallel  TimeDomain=Continuous-time  UseExternalTs=off  SampleTime=-1  IntegratorMethod=Forward Euler  FilterMethod=Forward Euler  ControllerParametersSource=internal  P=24/(Wtarget*n*Kpf)  I=1200  UseKiTs=off  D=0  UseExternalDerivativeSource=off  N=100  UseFilter=on  TunerSelectOption=Transfer Function Based (PID Tuner App)  InitialConditionSource=internal  InitialConditionForIntegrator=0  InitialConditionForFilter=0  DifferentiatorICPrevScaledInput=0  ExternalReset=none  TrackingMode=off  Kt=1  LimitOutput=off  SatLimitsSource=internal  UpperSaturationLimit=24  LowerSaturationLimit=0  LinearizeAsGain=on  AntiWindupMode=none  Kb=1  LimitIntegrator=off  UpperIntegratorSaturationLimit=inf  LowerIntegratorSaturationLimit=-inf  POutMin=[]  POutMax=[]  IOutMin=[]  IOutMax=[]  DOutMin=[]  DOutMax=[]  NOutMin=[]  NOutMax=[]  SumOutMin=[]  SumOutMax=[]  SaturationOutMin=[]  SaturationOutMax=[]  PParamMin=[]  PParamMax=[]  IParamMin=[]  IParamMax=[]  DParamMin=[]  DParamMax=[]  NParamMin=[]  NParamMax=[]  KbParamMin=[]  KbParamMax=[]  KtParamMin=[]  KtParamMax=[]  KbOutMin=[]  KbOutMax=[]  KtOutMin=[]  KtOutMax=[]  IntegratorOutMin=[]  IntegratorOutMax=[]  FilterOutMin=[]  FilterOutMax=[]  SumI1OutMin=[]  SumI1OutMax=[]  SumI2OutMin=[]  SumI2OutMax=[]  SumI3OutMin=[]  SumI3OutMax=[]  SumI4OutMin=[]  SumI4OutMax=[]  SumDOutMin=[]  SumDOutMax=[]  DifferentiatorOutMin=[]  DifferentiatorOutMax=[]  FilterDiffOutCoefMin=[]  FilterDiffOutCoefMax=[]  ReciprocalOutMin=[]  ReciprocalOutMax=[]  SumDenOutMin=[]  SumDenOutMax=[]  SumNumOutMin=[]  SumNumOutMax=[]  DivideOutMin=[]  DivideOutMax=[]  UdiffTsProdOutMin=[]  UdiffTsProdOutMax=[]  NTsProdOutMin=[]  NTsProdOutMax=[]  UintegralTsProdOutMin=[]  UintegralTsProdOutMax=[]  UngainTsProdOutMin=[]  UngainTsProdOutMax=[]  ClampingZeroOutDataTypeStr=Inherit: Inherit via back propagation  ClampingZeroOutMin=[]  ClampingZeroOutMax=[]  FilterDenConstantOutDataTypeStr=Inherit: Inherit via back propagation  FilterDenConstantOutMin=[]  FilterDenConstantOutMax=[]  PCopyOutDataTypeStr=Inherit: Inherit via back propagation  PCopyOutMin=[]  PCopyOutMax=[]  NCopyOutDataTypeStr=Inherit: Inherit via back propagation  NCopyOutMin=[]  NCopyOutMax=[]  IntegratorContinuousStateAttributes=''  IntegratorStateMustResolveToSignalObject=off  IntegratorRTWStateStorageClass=Auto  FilterContinuousStateAttributes=''  FilterStateMustResolveToSignalObject=off  FilterRTWStateStorageClass=Auto  ParallelPVariant=InternalParameters  IdealPVariant=Disabled  IVariant=InternalParameters  DVariant=Disabled  IntegratorVariant=Continuous  SatVariant=Disabled  AWVariant=Passthrough  PCopyVariant=Disabled  TRVariant=Disabled  FdbkBlocksVariant=Forward  IdealPFdbkVariant=Disabled  SatFdbkVariant=Disabled  DerivativeFilterVariant=Disabled  NVariant=Disabled  NCopyVariant=Disabled_SignalSpec  FilterICVariant=Disabled  IntegratorICVariant=InternalICs  ExternalResetVariant=Disabled  TRSumVariant=Passthrough  SumFdbkVariant=Disabled  SumVariant=Sum_PI  TsampFilterVariant=InternalTs  TsampNgainVariant=Passthrough  TsampIntegralVariant=Disabled_SignalSpec  ExternalSaturationOutDataTypeStr=Inherit: Same as second input  DerivativeSourceVariant=Disabled  PreIntVariant=InternalPreInt
  Selector : Selector  InputPortWidth=4  IndexOptions=Index vector (dialog)  Indices=2  OutputSizes=1
  Selector1 : Selector  InputPortWidth=4  IndexOptions=Index vector (dialog)  Indices=4  OutputSizes=1
  Selector2 : Selector  InputPortWidth=4  IndexOptions=Index vector (dialog)  Indices=3  OutputSizes=1
  State-Space : StateSpace  A=A_Task8  B=B_Task8  C=C_Task8  D=D_Task8  InitialCondition=0
  Stop Simulation : Stop
  Subtract : Sum  Inputs=+-
  Sum : Sum  Inputs=|+-
  Switch : Switch  Threshold=23.8  SaturateOnIntegerOverflow=off  InputSameDT=off
  Terminator : Terminator
  Terminator1 : Terminator
  wires:
  Integrator/1 -> Gain8/1  "I_t_Task_11"
  Subtract/1 -> Gain5/1
  Gain8/1 -> Terminator/1  "Ih_Task_11"
  Gain9/1 -> Add/4
  Gain3/1 -> Sum/1
  Switch/1 -> Stop Simulation/1
  Selector2/1 -> Sum/2, Gain7/1
  Gain/1 -> Add/3
  Gain2/1 -> Add/2
  Gain4/1 -> Gain6/1
  Gain5/1 -> Integrator/1  "I_Task_11"
  Selector/1 -> Gain/1, Gain4/1
  Gain7/1 -> Subtract/2
  Constant1/1 -> Switch/1
  PID Controller/1 -> State-Space/1, Subtract/1  "v_task11"
  Gain1/1 -> Add/1
  Add/1 -> Switch/2
  State-Space/1 -> Selector2/1, Selector/1, Selector1/1  "States Task11"
  Derivative/1 -> Gain2/1
  Gain6/1 -> Gain9/1, Terminator1/1
  Constant/1 -> Switch/3
  Sum/1 -> PID Controller/1
  Selector1/1 -> Derivative/1, Gain1/1
  Constant2/1 -> Gain3/1  "ref"

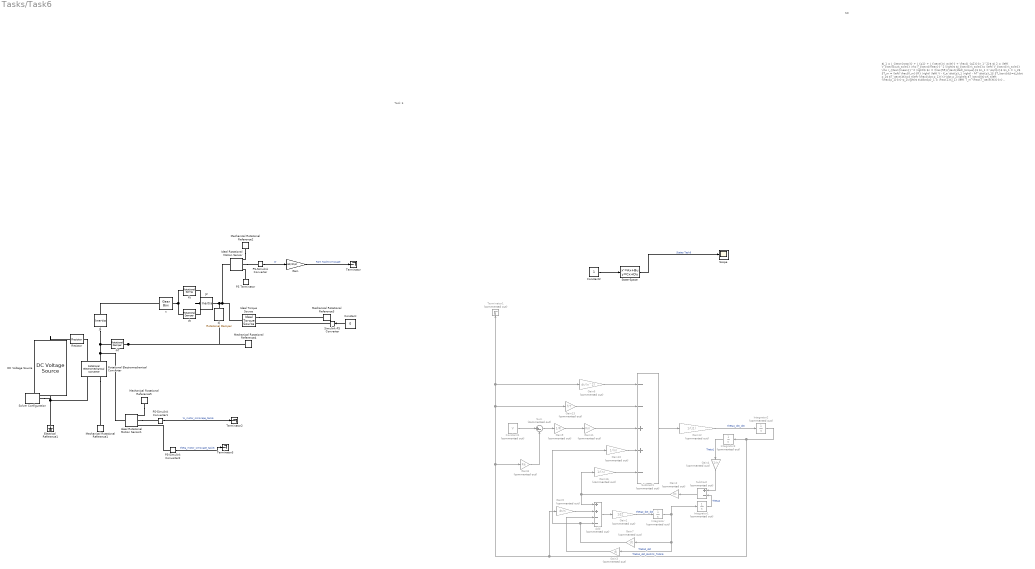
== system Tasks/Task6  ==
  note: $J_1 = J_{\text{rotor}} + J_{g1} + J_{\text{in\_axle}} + \frac{J_{g2}}{n_1^2}$
      | $J_2 = \left( V_{\text{out\_axle}} \rho r_{\text{mean}}^2 \right)$
      |
      | $J_{\text{in\_axle}}= \left( V_{\text{in\_axle}} \rho r_{\text{mean}}^2 \right)$
      |
      | $n = \frac{55}{\text{stall\_torque}}$
      | $n_1 = \sqrt{n}$
      | $n_1 = n_2$
      |
      | $T_m = \left( \frac{K_m}{R} \right) \left( V - K_e \dot{p}_1 \right) - frT \dot{p}_1$
      | $T_\text{dj}=d_j\dot p_2$
      | $T_\text{dt}=d_t\left (\frac{\dot p_1}{n}-\dot p_2\right)$
      | $T_\text{Kt}=K_t\left (\frac{p_1}{n}-p_2\right)$
      |
      | $\ddot{p}_1 = \frac{1}{J_1} \left( T_m -\frac{T_\text{Kt}}{n} -\frac{T_\text{dt}}{n}\right)$
      |
      | $\ddot{p}_1 = \frac{1}{J_1} \left( \frac{K_mV}{R} - \frac{K_t}{n^2}p_1 -\frac{K_t}{n} p_2 - \left(\frac{d_t}{n^2} -\frac{K_mK_e}{R}- frT\right)\dot{p}_1 +\frac{dt}{n}\dot{p}_2\right)$
      | $\ddot{p}_2 = \frac{1}{J_2} \left(T_\text{Kt} +T_\text{dt}-T_\text{dj}\right)$
      | $\ddot{p}_2 = \frac{1}{J_2} \left( K_t\frac{p_1}{n} - K_t p_2 +\frac{dt}{n}\dot{p}_1 - (d_j+d_t)\dot{p}_2\right)$
  note: Task 6
  note: SD
  Add : Sum  Commented=on  Inputs=++--
  Constant : Constant  Value=0
  Constant1 : Constant  Commented=on  Value=V
  Constant2 : Constant
  DC Voltage Source : fl_lib/Electrical/Electrical Sources/DC Voltage Source  v0=V V
  Electrical Reference1 : fl_lib/Electrical/Electrical Elements/Electrical Reference
  Gain : Gain  Gain=60/(2*pi)
  Gain1 : Gain  Commented=on  Gain=1/J2
  Gain10 : Gain  Commented=on  Gain=1/(n)
  Gain11 : Gain  Commented=on  Gain=Km
  Gain12 : Gain  Commented=on  Gain=1/(J1)
  Gain13 : Gain  Commented=on  Gain=frT
  Gain16 : Gain  Commented=on  Gain=1/(n)
  Gain2 : Gain  Commented=on  Gain=Kt
  Gain3 : Gain  Commented=on  Gain=dj
  Gain4 : Gain  Commented=on  Gain=1/n
  Gain5 : Gain  Commented=on  Gain=dt/n
  Gain6 : Gain  Commented=on  Gain=dt/(n^2)
  Gain7 : Gain  Commented=on  Gain=dt
  Gain8 : Gain  Commented=on  Gain=Ke
  Gain9 : Gain  Commented=on  Gain=1/R
  Ideal Rotational Motion Sensor : fl_lib/Mechanical/Mechanical Sensors/Ideal Rotational Motion Sensor  reference=foundation.enum.MeasurementReference.difference  acceleration_port=false  velocity_port=true  position_port=true  wrap_angle=simscape.enum.onoff.off  offset=0 rad
  Ideal Rotational Motion Sensor1 : fl_lib/Mechanical/Mechanical Sensors/Ideal Rotational Motion Sensor  reference=foundation.enum.MeasurementReference.difference  acceleration_port=false  velocity_port=true  position_port=true  wrap_angle=simscape.enum.onoff.off  offset=0 rad
  Ideal Torque Source : fl_lib/Mechanical/Mechanical Sources/Ideal Torque Source
  Integrator{,1..3} (4 alike) : Integrator  Commented=on
  J1 : fl_lib/Mechanical/Rotational Elements/Inertia  inertia=J1 kg*m^2  num_ports=foundation.enum.numPorts2.two  w_specify=off  w_priority=High  w=0 rad/s  w_nominal_specify=off  w_nominal_value=1  w_nominal_unit=rad/s  t_specify=off  t_priority=None  t=0 N*m  t_nominal_specify=off  t_nominal_value=1  t_nominal_unit=N*m
      settings: InternalSimscapePortConfiguration="{\"Bottom\":[],\"Left\":[{\"id\":\"I\",\"label\":\"\",\"type\":\"foundation.mechanical.rotational.rotational\"}],\"Right\":[{\"id\":\"J\",\"label\":\"\",\"type\":\"foundation.mechanical.rotational.rotational\"}],\"Top\":[]}"
  J2 : fl_lib/Mechanical/Rotational Elements/Inertia  inertia=J2 kg*m^2  num_ports=foundation.enum.numPorts2.two  w_specify=off  w_priority=High  w=0 rad/s  w_nominal_specify=off  w_nominal_value=1  w_nominal_unit=rad/s  t_specify=off  t_priority=None  t=0 N*m  t_nominal_specify=off  t_nominal_value=1  t_nominal_unit=N*m
      settings: InternalSimscapePortConfiguration="{\"Bottom\":[],\"Left\":[{\"id\":\"I\",\"label\":\"\",\"type\":\"foundation.mechanical.rotational.rotational\"}],\"Right\":[{\"id\":\"J\",\"label\":\"\",\"type\":\"foundation.mechanical.rotational.rotational\"}],\"Top\":[]}"
  Kt : fl_lib/Mechanical/Rotational Elements/Rotational Spring  spr_rate=Kt N*m/rad  w_specify=off  w_priority=None  w=0 rad/s  w_nominal_specify=off  w_nominal_value=1  w_nominal_unit=rad/s  t_specify=off  t_priority=None  t=0 N*m  t_nominal_specify=off  t_nominal_value=1  t_nominal_unit=N*m  phi_specify=off  phi_priority=High  phi=0 rad  phi_nominal_specify=off  phi_nominal_value=1  phi_nominal_unit=rad
  Mechanical Rotational Reference{1..5} (5 alike) : fl_lib/Mechanical/Rotational Elements/Mechanical Rotational Reference
  PS Terminator : fl_lib/Physical Signals/Sinks/PS Terminator
  PS-Simulink Converter : nesl_utility/PS-Simulink Converter  PhysicalDomain=network_engine_domain  SubClassName=ps_output  LeftPortType=input  RightPortType=output  PseudoPeriodic=off  Frequencies=[]  VectorFormat=inherit  Unit=inherit  AffineConversion=off
  PS-Simulink Converter1 : nesl_utility/PS-Simulink Converter  PhysicalDomain=network_engine_domain  SubClassName=ps_output  LeftPortType=input  RightPortType=output  PseudoPeriodic=off  Frequencies=[]  VectorFormat=inherit  Unit=inherit  AffineConversion=off
  PS-Simulink Converter2 : nesl_utility/PS-Simulink Converter  PhysicalDomain=network_engine_domain  SubClassName=ps_output  LeftPortType=input  RightPortType=output  PseudoPeriodic=off  Frequencies=[]  VectorFormat=inherit  Unit=inherit  AffineConversion=off
  Resistor : fl_lib/Electrical/Electrical Elements/Resistor  R=R Ohm  i_specify=off  i_priority=None  i=0 A  i_nominal_specify=off  i_nominal_value=1  i_nominal_unit=A  v_specify=off  v_priority=None  v=0 V  v_nominal_specify=off  v_nominal_value=1  v_nominal_unit=V
  Rotational Electromechanical Converter : fl_lib/Electrical/Electrical Elements/Rotational Electromechanical Converter  K=Ke V*s/rad  i_specify=off  i_priority=None  i=0 A  i_nominal_specify=off  i_nominal_value=1  i_nominal_unit=A  v_specify=off  v_priority=None  v=0 V  v_nominal_specify=off  v_nominal_value=1  v_nominal_unit=V  t_specify=off  t_priority=None  t=0 N*m  t_nominal_specify=off  t_nominal_value=1  t_nominal_unit=N*m  w_specify=on  w_priority=None  w=0 rad/s  w_nominal_specify=off  w_nominal_value=1  w_nominal_unit=rad/s
  Scope : Scope
  Simulink-PS Converter : nesl_utility/Simulink-PS Converter  PhysicalDomain=network_engine_domain  SubClassName=ps_input  LeftPortType=input  RightPortType=output  PseudoPeriodic=off  Frequencies=[]  NoiseDistribution=none  NoiseParameters=[]  Unit=1  AffineConversion=off  FilteringAndDerivatives=provide  SimscapeFilterOrder=1  InputFilterTimeConstant=0.001  UdotUserProvided=0
  Solver Configuration : nesl_utility/Solver Configuration  PhysicalDomain=network_engine_domain  SubClassName=solver  LeftPortType=input  RightPortType=generic  Tones=[]  Harmonics=[]  SimulateNoise=off  Profile=off  UseLocalSampling=off  EnableSwitchedLinearOptims=on  FrequencyDomain=off  UseCCode=off  RelTol=0.001  AbsTol=0.001  MinStep=1e-09  ToWorkspace=off  RevertToSquareIcSolve=off  NumHomotopyIterations=100  PhasorMode=off  PhasorModeNumHarmonics=1  ConsistencySolver=NEWTON_FTOL  IndexReductionMethod=DerivativeReplacement  DoDC=off  ResidualTolerance=1e-09  ConsistencyTolSource=GLOBAL  ConsistencyAbsTol=0.001  ConsistencyRelTol=0.001  ConsistencyTolFactor=0.001  UseLocalSolver=off  LocalSolverChoice=NE_BACKWARD_EULER_ADVANCER  ResolveIndetEquations=on  FunctionEvalNumThread=1  LocalSolverSampleTime=0.001  DoFixedCost=off  MaxNonlinIter=3  MaxModeIter=2  ComputeImpulses=off  ImpulseIterations=2  LinearAlgebra=auto  LinearAlgebraNumThread=0  EquationFormulation=NE_TIME_EF  DelaysMemoryBudget=1024  AutomaticFiltering=on  FilteringTimeConstant=0.001  PartitionStorageMethod=AS_NEEDED  PartitionMemoryBudget=1024  PartitionMethod=ROBUST  MultibodyUseLocalSolver=off  MultibodyLocalSolverChoice=ODE1  MultibodyLocalSolverSampleTime=0.001
  State-Space : StateSpace  A=A_Task6  B=B_Task6  C=C_Task6  D=D_Task6  InitialCondition=0
  Subtract : Sum  Commented=on  Inputs=+-
  Subtract1 : Sum  Commented=on  Inputs=--++-
  Sum : Sum  Commented=on  Inputs=|+-
  Terminator : Terminator
  Terminator1 : Terminator  Commented=on
  Terminator2 : Terminator
  Terminator3 : Terminator
  dj : fl_lib/Mechanical/Rotational Elements/Rotational Damper  D=dj N*m*s/rad  w_specify=off  w_priority=None  w=0 rad/s  w_nominal_specify=off  w_nominal_value=1  w_nominal_unit=rad/s  t_specify=off  t_priority=None  t=0 N*m  t_nominal_specify=off  t_nominal_value=1  t_nominal_unit=N*m
  dt : fl_lib/Mechanical/Rotational Elements/Rotational Damper  D=dt N*m*s/rad  w_specify=off  w_priority=None  w=0 rad/s  w_nominal_specify=off  w_nominal_value=1  w_nominal_unit=rad/s  t_specify=off  t_priority=None  t=0 N*m  t_nominal_specify=off  t_nominal_value=1  t_nominal_unit=N*m
  frT : fl_lib/Mechanical/Rotational Elements/Rotational Damper  D=frT N*m*s/rad  w_specify=off  w_priority=None  w=0 rad/s  w_nominal_specify=off  w_nominal_value=1  w_nominal_unit=rad/s  t_specify=off  t_priority=None  t=0 N*m  t_nominal_specify=off  t_nominal_value=1  t_nominal_unit=N*m
  n : fl_lib/Mechanical/Mechanisms/Gear Box  ratio=n  t_in_specify=off  t_in_priority=None  t_in=0 N*m  t_in_nominal_specify=off  t_in_nominal_value=1  t_in_nominal_unit=N*m  t_out_specify=off  t_out_priority=None  t_out=0 N*m  t_out_nominal_specify=off  t_out_nominal_value=1  t_out_nominal_unit=N*m
  wires:
  PS-Simulink Converter/1 -> Gain/1  "W"
  Gain/1 -> Terminator/1  "Rpm Task5 simscape"
  Constant/1 -> Simulink-PS Converter/1
  Gain4/1 -> Subtract/1
  Subtract/1 -> Gain2/1
  Gain16/1 -> Subtract1/5
  Gain12/1 -> Integrator2/1  "theta1_dot_dot"
  Add/1 -> Gain1/1
  Sum/1 -> Gain9/1
  Gain9/1 -> Gain11/1
  Integrator2/1 -> Gain5/1, Terminator1/1, Gain6/1, Gain13/1, Gain8/1, Integrator3/1  "Theta1_dot_BLOCK_TASK6"
  Integrator3/1 -> Gain4/1  "Theta1"
  Gain13/1 -> Subtract1/2
  Integrator1/1 -> Subtract/2  "Theta2"
  Subtract1/1 -> Gain12/1
  Integrator/1 -> Integrator1/1, Gain7/1, Gain3/1  "Theta2_dot"
  Gain11/1 -> Subtract1/3
  Constant1/1 -> Sum/1
  Gain3/1 -> Add/3
  Gain1/1 -> Integrator/1  "theta2_dot_dot"
  Gain8/1 -> Sum/2
  PS-Simulink Converter1/1 -> Terminator2/1  "W_motor_simscape_task6"
  Gain6/1 -> Subtract1/1
  Constant2/1 -> State-Space/1
  State-Space/1 -> Scope/1  "States Task6"
  PS-Simulink Converter2/1 -> Terminator3/1  "theta_motor_simscape_task6"
  Gain5/1 -> Add/2
  Gain7/1 -> Add/4, Gain10/1
  Gain2/1 -> Gain16/1, Add/1
  Gain10/1 -> Subtract1/4
  connections:
  Ideal Rotational Motion Sensor/RConn2 -- PS-Simulink Converter/LConn1
  Resistor/RConn1 -- Rotational Electromechanical Converter/LConn1
  Rotational Electromechanical Converter/RConn2 -- Mechanical Rotational Reference1/LConn1
  Ideal Torque Source/RConn2 -- Mechanical Rotational Reference3/LConn1
  frT/RConn1 -- Mechanical Rotational Reference4/LConn1 -- dj/RConn1
  PS Terminator/LConn1 -- Ideal Rotational Motion Sensor/RConn3
  DC Voltage Source/LConn1 -- Resistor/LConn1
  n/RConn1 -- dt/LConn1 -- Kt/LConn1
  J2/RConn1 -- dj/LConn1 -- Ideal Rotational Motion Sensor/LConn1 -- Ideal Torque Source/LConn1
  Simulink-PS Converter/RConn1 -- Ideal Torque Source/RConn1
  PS-Simulink Converter2/LConn1 -- Ideal Rotational Motion Sensor1/RConn3
  Ideal Rotational Motion Sensor1/RConn2 -- PS-Simulink Converter1/LConn1
  J2/LConn1 -- dt/RConn1 -- Kt/RConn1
  J1/LConn1 -- n/LConn1
  Rotational Electromechanical Converter/LConn2 -- Ideal Rotational Motion Sensor1/LConn1 -- frT/LConn1 -- J1/RConn1
  Electrical Reference1/LConn1 -- Rotational Electromechanical Converter/RConn1 -- Solver Configuration/RConn1 -- DC Voltage Source/RConn1
  Mechanical Rotational Reference2/LConn1 -- Ideal Rotational Motion Sensor/RConn1
  Mechanical Rotational Reference5/LConn1 -- Ideal Rotational Motion Sensor1/RConn1

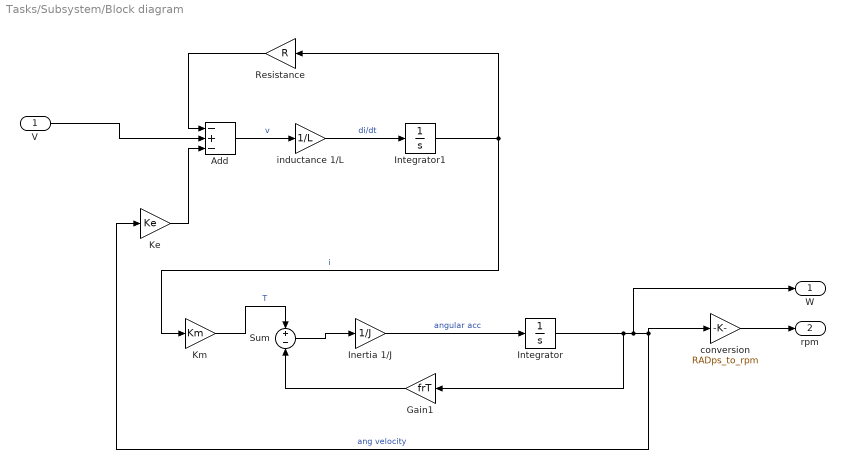
== system Tasks/Subsystem/Block diagram ==
  V : Inport
  Add : Sum  Inputs=-+-
  Gain1 : Gain  Gain=frT
  Inertia 1/J : Gain  Gain=1/J
  Integrator : Integrator
  Integrator1 : Integrator
  Ke : Gain  Gain=Ke
  Km : Gain  Gain=Km
  Resistance : Gain  Gain=R
  Sum : Sum  Inputs=+-
  conversion : Gain  Gain=RADps_to_rpm
  inductance 1/L : Gain  Gain=1/L
  W : Outport
  rpm : Outport  Port=2
  wires:
  Ke/1 -> Add/3
  Sum/1 -> Inertia 1/J/1
  inductance 1/L/1 -> Integrator1/1  "di/dt"
  Km/1 -> Sum/1  "T"
  Inertia 1/J/1 -> Integrator/1  "angular acc"
  Gain1/1 -> Sum/2
  Add/1 -> inductance 1/L/1  "v"
  Integrator1/1 -> Km/1, Resistance/1  "i"
  Integrator/1 -> conversion/1, Ke/1, W/1, Gain1/1  "ang velocity"
  Resistance/1 -> Add/1
  V/1 -> Add/2
  conversion/1 -> rpm/1

== system Tasks/Subsystem/PI controller ==
  note: Develop in Simulink an angular velocity PI controller for the DC-motor using the block-diagram model of the motor and show the resulting block diagram model. Assume that you can sense angular velocity and acceleration directly. Tune the controller to make a quick response without overshooting to an input reference step of 12 rad/s and make sure and demonstrate not to violate any voltage or current limitations of the motor. However, the starting current is allowed to be 500% of the rated current. Demonstrate the controller’s performance by time domain plots and state your controller settings
  ang velocity : Inport
  Step : Step  Time=0  After=12  SampleTime=0
  Sum1 : Sum  Inputs=+-
  Varying PID Controller : slpidlib/PID Controller  Controller=PI  Form=Parallel  TimeDomain=Continuous-time  UseExternalTs=off  SampleTime=-1  IntegratorMethod=Forward Euler  FilterMethod=Forward Euler  ControllerParametersSource=internal  P=0.218326262588512  I=6.46147954848858  UseKiTs=off  D=0  UseExternalDerivativeSource=off  N=100  UseFilter=on  TunerSelectOption=Transfer Function Based (PID Tuner App)  InitialConditionSource=internal  InitialConditionForIntegrator=0  InitialConditionForFilter=0  DifferentiatorICPrevScaledInput=0  ExternalReset=none  TrackingMode=off  Kt=1  LimitOutput=on  SatLimitsSource=internal  UpperSaturationLimit=V*1.2  LowerSaturationLimit=0  LinearizeAsGain=off  AntiWindupMode=none  Kb=1  LimitIntegrator=off  UpperIntegratorSaturationLimit=inf  LowerIntegratorSaturationLimit=-inf  POutMin=[]  POutMax=[]  IOutMin=[]  IOutMax=[]  DOutMin=[]  DOutMax=[]  NOutMin=[]  NOutMax=[]  SumOutMin=[]  SumOutMax=[]  SaturationOutMin=[]  SaturationOutMax=[]  PParamMin=[]  PParamMax=[]  IParamMin=[]  IParamMax=[]  DParamMin=[]  DParamMax=[]  NParamMin=[]  NParamMax=[]  KbParamMin=[]  KbParamMax=[]  KtParamMin=[]  KtParamMax=[]  KbOutMin=[]  KbOutMax=[]  KtOutMin=[]  KtOutMax=[]  IntegratorOutMin=[]  IntegratorOutMax=[]  FilterOutMin=[]  FilterOutMax=[]  SumI1OutMin=[]  SumI1OutMax=[]  SumI2OutMin=[]  SumI2OutMax=[]  SumI3OutMin=[]  SumI3OutMax=[]  SumI4OutMin=[]  SumI4OutMax=[]  SumDOutMin=[]  SumDOutMax=[]  DifferentiatorOutMin=[]  DifferentiatorOutMax=[]  FilterDiffOutCoefMin=[]  FilterDiffOutCoefMax=[]  ReciprocalOutMin=[]  ReciprocalOutMax=[]  SumDenOutMin=[]  SumDenOutMax=[]  SumNumOutMin=[]  SumNumOutMax=[]  DivideOutMin=[]  DivideOutMax=[]  UdiffTsProdOutMin=[]  UdiffTsProdOutMax=[]  NTsProdOutMin=[]  NTsProdOutMax=[]  UintegralTsProdOutMin=[]  UintegralTsProdOutMax=[]  UngainTsProdOutMin=[]  UngainTsProdOutMax=[]  ClampingZeroOutDataTypeStr=Inherit: Inherit via back propagation  ClampingZeroOutMin=[]  ClampingZeroOutMax=[]  FilterDenConstantOutDataTypeStr=Inherit: Inherit via back propagation  FilterDenConstantOutMin=[]  FilterDenConstantOutMax=[]  PCopyOutDataTypeStr=Inherit: Inherit via back propagation  PCopyOutMin=[]  PCopyOutMax=[]  NCopyOutDataTypeStr=Inherit: Inherit via back propagation  NCopyOutMin=[]  NCopyOutMax=[]  IntegratorContinuousStateAttributes=''  IntegratorStateMustResolveToSignalObject=off  IntegratorRTWStateStorageClass=Auto  FilterContinuousStateAttributes=''  FilterStateMustResolveToSignalObject=off  FilterRTWStateStorageClass=Auto  ParallelPVariant=InternalParameters  IdealPVariant=Disabled  IVariant=InternalParameters  DVariant=Disabled  IntegratorVariant=Continuous  SatVariant=Enabled  AWVariant=Passthrough  PCopyVariant=Disabled  TRVariant=Disabled  FdbkBlocksVariant=Forward  IdealPFdbkVariant=Disabled  SatFdbkVariant=Disabled  DerivativeFilterVariant=Disabled  NVariant=Disabled  NCopyVariant=Disabled_SignalSpec  FilterICVariant=Disabled  IntegratorICVariant=InternalICs  ExternalResetVariant=Disabled  TRSumVariant=Passthrough  SumFdbkVariant=Disabled  SumVariant=Sum_PI  TsampFilterVariant=InternalTs  TsampNgainVariant=Passthrough  TsampIntegralVariant=Disabled_SignalSpec  ExternalSaturationOutDataTypeStr=Inherit: Same as second input  DerivativeSourceVariant=Disabled  PreIntVariant=InternalPreInt
  V : Outport
  wires:
  Sum1/1 -> Varying PID Controller/1
  Step/1 -> Sum1/1
  ang velocity/1 -> Sum1/2  "Feedback_PI"
  Varying PID Controller/1 -> V/1  "PI_output"
